simulink model "B6_Buck"  (R2022a)
settings: Solver=ode23tb  StartTime=0.0  StopTime=0.2  MaxStep=1e-2  RelTol=1e-4
values from neighbouring files (symbols this model uses):
  Schaltfrequenz = 20e3    (= 20000)    [Config.m]
undefined symbols (not defined in the file or in its folder): plecs
settings Model: SimulationMode=accelerator  Creator=sisfort  LastModifiedBy=jheinemann
settings SolverCC: MaxConsecutiveZCs=100000000  SolverResetMethod=Robust  AutoInsertRateTranBlk=on
settings DebuggingCC: UnconnectedInputMsg=warning  UnconnectedOutputMsg=warning  UnconnectedLineMsg=warning
settings RTWCC: DLArmComputeVersion=19.05

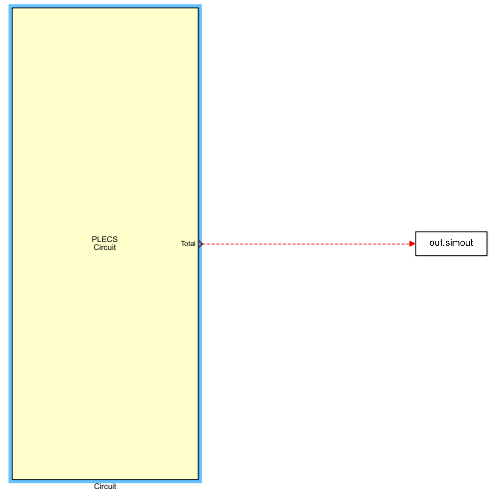
[thumbnail: Simulink's stored preview of the top-level diagram]
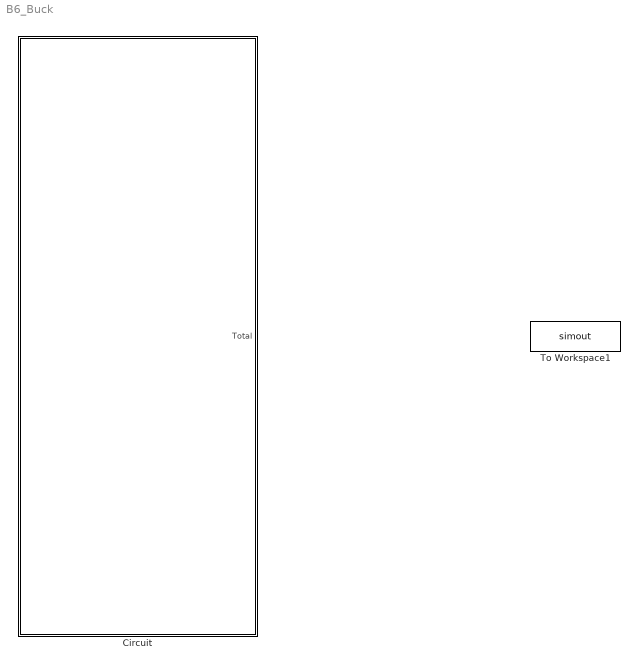
== system B6_Buck ==
  Circuit : Subsystem  LoadFcn=plecs('sl', 200);  InitFcn=plecs('sl', 214);  StartFcn=plecs('sl', 208);  StopFcn=plecs('sl', 209);  mask(PlecsCircuit){PLECSData=<binary blob, 29440 chars, not shown>}
      mask prompts: PLECSData "PLECS Data (Do not delete or modify!)"
      mask init:
      | % PLACE CUSTOM INITIALIZATIONS ABOVE
      | % DO NOT REMOVE
      | plecs('sl', 215);
      | % DO NOT REMOVE
      settings: CopyFcn=plecs('sl', 203);  DeleteFcn=plecs('sl', 205);  UndoDeleteFcn=plecs('sl', 206);  PreSaveFcn=plecs('sl', 211);  PostSaveFcn=plecs('sl', 201);  NameChangeFcn=plecs('sl', 210);  DestroyFcn=plecs('sl', 207);  PreCopyFcn=plecs('sl', 216);  OpenFcn=plecs('sl', 202);  ErrorFcn=plerrorfcn
      mask Help: web(['file:///' fullfile(plecsdoc, 'creatingacircuit.html')])
      mask Display: disp('PLECS\nCircuit')
  To Workspace1 : ToWorkspace  VariableName=simout  SampleTime=1/(Schaltfrequenz*10)
      settings: MaxDataPoints=1/50*3*Schaltfrequenz*10
  wires:
  ? -> To Workspace1/1

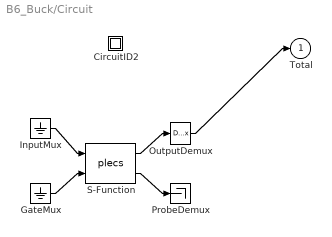
== system B6_Buck/Circuit ==
  " CircuitID2 " : Subsystem
  " GateMux " : Ground
  " InputMux " : Ground
  " OutputDemux " : Demux  Outputs=[ 48 ]
  " ProbeDemux " : Terminator
  " S-Function " : S-Function  FunctionName=plecs  SFunctionDeploymentMode=off  EnableBusSupport=off
  Total : Outport  PortDimensions=48
  wires:
  " InputMux "/1 -> " S-Function "/1
  " GateMux "/1 -> " S-Function "/2
  " S-Function "/1 -> " OutputDemux "/1
  " S-Function "/2 -> " ProbeDemux "/1
  " OutputDemux "/1 -> Total/1

== system B6_Buck/Circuit/ CircuitID2  ==
